simulink model "Control_Subscribe"  (R2018b)
settings: Solver=VariableStepAuto  StartTime=0.0  StopTime=inf  RelTol=1e-3
libraries: robotlib x1
settings Model: Creator=mskim  LastModifiedBy=mskim

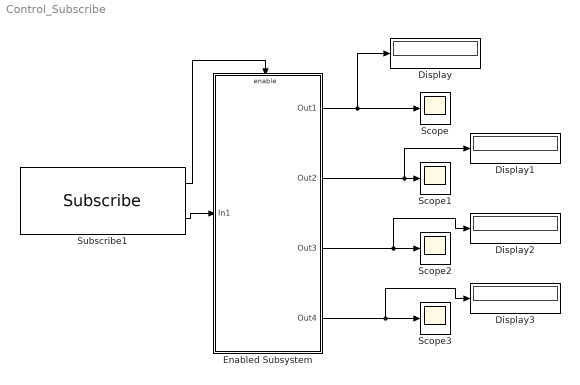
== system Control_Subscribe ==
  Display{,1..3} (4 alike) : Display
  Enabled Subsystem : Subsystem
  Scope{,1..3} (4 alike) : Scope
  Subscribe1 : robotlib/Subscribe  topicSource=Specify your own  topic=/my_msgs/ControlCommand  messageType=my_msgs/ControlCommand  sampleTime=-1  messageQueueLength=51
      settings: SourceProductBaseCode=RO
  wires:
  Subscribe1/2 -> Enabled Subsystem/1(In1)
  Subscribe1/1 -> Enabled Subsystem/Enable
  Enabled Subsystem/1(Out1) -> Display/1, Scope/1
  Enabled Subsystem/2(Out2) -> Display1/1, Scope1/1
  Enabled Subsystem/3(Out3) -> Display2/1, Scope2/1
  Enabled Subsystem/4(Out4) -> Display3/1, Scope3/1

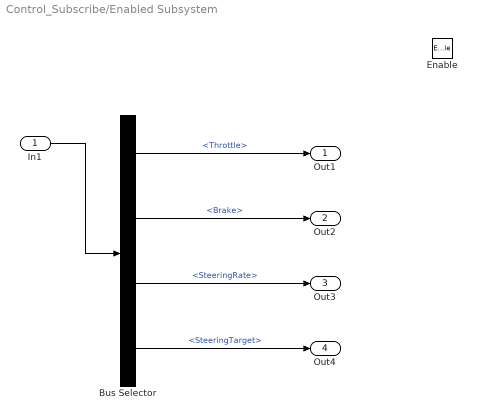
== system Control_Subscribe/Enabled Subsystem ==
  In1 : Inport
  Enable : EnablePort
  Bus Selector : BusSelector  DialogController=Simulink.DDGSource_BusSelector  OutputSignals=Throttle,Brake,SteeringRate,SteeringTarget
  Out1 : Outport
  Out2 : Outport  Port=2
  Out3 : Outport  Port=3
  Out4 : Outport  Port=4
  wires:
  In1/1 -> Bus Selector/1
  Bus Selector/1 -> Out1/1  "<Throttle>"
  Bus Selector/2 -> Out2/1  "<Brake>"
  Bus Selector/3 -> Out3/1  "<SteeringRate>"
  Bus Selector/4 -> Out4/1  "<SteeringTarget>"
